simulink model "Wind_Turbine_Fixed_Speed_AC_to_DC_Output"  (R2019b)
settings: Solver=ode4  StartTime=0.0  StopTime=10  FixedStep=10e-6  RelTol=1e-3
libraries: powerlib x16, powerlib_meascontrol x5, re_lib x1, simulink x1
settings Model: Creator=KUNAL  LastModifiedBy=KUNAL

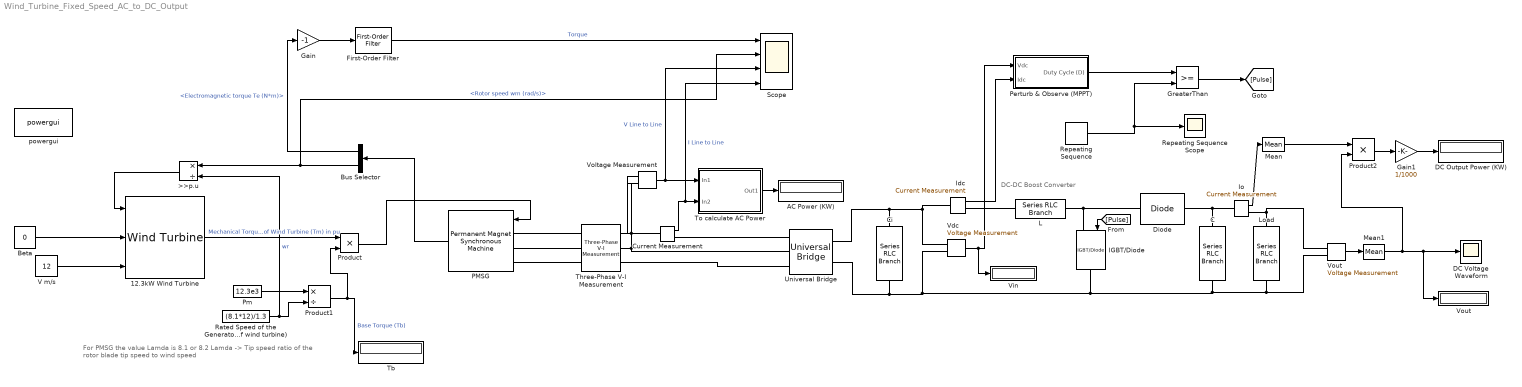
== system Wind_Turbine_Fixed_Speed_AC_to_DC_Output ==
  note: For PMSG the value Lamda is 8.1 or 8.2
      | Lamda -> Tip speed ratio of the rotor blade tip speed to wind speed
  note: DC-DC Boost Converter
  12.3kW Wind Turbine : re_lib/Wind Generation/Wind Turbine  Pnom=12.3e3  Pelec_base=12.3e3/0.9  wind_base=12  P_wind_base=0.85  speed_nom=1.2  pitch_angle=0  c1_c6="[0.51763          116          0.4            5           21     0.006795]"  cp_nom=0.48  lambda_nom=8.1
      settings: SourceProductName=Simscape Electrical  SourceProductBaseCode=PS
  ">>p.u " : Product  Inputs=*/
  "AC Power (KW) " : Display
  Beta : Constant  Value=0
  Bus Selector : BusSelector  OutputSignals=Electromagnetic torque Te (N*m),Rotor speed wm (rad/s)
  C : powerlib/Elements/Series RLC Branch  LConnTagsString=__new0  RConnTagsString=__new0  BranchType=C  Resistance=0.005  Inductance=1e-3  SetiL0=off  InitialCurrent=0  Capacitance=6.6094e-04  Setx0=off  InitialVoltage=0  Measurements=None
      settings: SourceProductName=Simscape Electrical
  "Ci " : powerlib/Elements/Series RLC Branch  LConnTagsString=__new0  RConnTagsString=__new0  BranchType=RC  Resistance=0.005  Inductance=1e-3  SetiL0=off  InitialCurrent=0  Capacitance=500e-6  Setx0=off  InitialVoltage=0  Measurements=None
      settings: SourceProductName=Simscape Electrical
  Current Measurement : powerlib/Measurements/Current Measurement  PhasorSimulation=off  OutputType=Complex  PSBequivalent=0
      settings: SourceProductName=Simscape Electrical
  "DC Output Power (KW) " : Display
  "DC Voltage Waveform " : Scope
  Diode : powerlib/Power Electronics/Diode  Ron=0.001  Lon=0  Vf=0.8  IC=0  UseSnubber=0  Rs=inf  Cs=inf  Measurements=off
      settings: SourceProductName=Simscape Electrical
  First-Order Filter : powerlib_meascontrol/Filters/First-Order Filter  FilterType=Lowpass  Tc=10e-3  Ts=50e-6  Initialize=on  Vac_Init=[0, 0, 50]  Vdc_Init=0  PlotResponse=off  FreqRange="[0,  200,  1]"
      settings: SourceProductName=Simscape Electrical
  Gain : Gain  Gain=-1
  Gain1 : Gain  Gain=1/1000
  GreaterThan : RelationalOperator  OutDataTypeStr=boolean  RndMeth=Simplest
  IGBT/Diode : powerlib/Power Electronics/IGBT//Diode  Ron=1e-3  Rs=1e5  Cs=inf  Measurements=off
      settings: SourceProductName=Simscape Electrical
  "Idc " : powerlib/Measurements/Current Measurement  PhasorSimulation=off  OutputType=Complex  PSBequivalent=0
      settings: SourceProductName=Simscape Electrical
  "Io " : powerlib/Measurements/Current Measurement  PhasorSimulation=off  OutputType=Complex  PSBequivalent=0
      settings: SourceProductName=Simscape Electrical
  "L " : powerlib/Elements/Series RLC Branch  LConnTagsString=__new0  RConnTagsString=__new0  BranchType=L  Resistance=0.005  Inductance=4.5573e-05  SetiL0=off  InitialCurrent=0  Capacitance=500e-6  Setx0=off  InitialVoltage=0  Measurements=None
      settings: SourceProductName=Simscape Electrical
  Load : powerlib/Elements/Series RLC Branch  LConnTagsString=__new0  RConnTagsString=__new0  BranchType=R  Resistance=13.5  Inductance=1e-3  SetiL0=off  InitialCurrent=0  Capacitance=500e-6  Setx0=off  InitialVoltage=0  Measurements=None
      settings: SourceProductName=Simscape Electrical
  Mean : powerlib_meascontrol/Measurements/Mean  Freq=60  Vinit=0  Ts=50e-6
      settings: SourceProductName=Simscape Electrical
  Mean1 : powerlib_meascontrol/Measurements/Mean  Freq=60  Vinit=0  Ts=50e-6
      settings: SourceProductName=Simscape Electrical
  "PMSG " : powerlib/Machines/Permanent Magnet Synchronous Machine  NbPhases=3  FluxDistribution=Sinusoidal  RotorType=Salient-pole  MechanicalLoad=Torque Tm  PresetModel=No  ShowDetailedParameters=on  MeasurementBus=off  Resistance=0.0485  Inductance=8.5e-3  dqInductances=[0.395e-3,0.395e-3]  La=0.000395  MachineConstant=Flux linkage established by magnets (V.s)  Flux=0.1194  VoltageCst=86.6271  TorqueCst=0.7164  Flat=120  Mechanical=[0.0027 0.0004924 4 0]  PolePairs=4  InitialConditions=[0,0, 0,0]  InitialConditions5ph=[0 0 0 0 0 0]  RefAngle=90 degrees behind phase A axis (modified Park)  IterativeDiscreteModel=Trapezoidal non iterative  TsBlock=-1  TsPowergui=0
  "Perturb & Observe (MPPT) " : Subsystem
  "Pm " : Constant  Value=12.3e3
  Product : Product  Inputs=**
  Product1 : Product  Inputs=*/
  Product2 : Product
  Rated Speed of the Generator (Wr) (Lamda * Wind Speed /Radius of wind turbine) : Constant  Value=(8.1*12)/1.3
  Repeating Sequence : simulink/Sources/Repeating Sequence  rep_seq_t=[0 1/20000]  rep_seq_y=[0 0.9]
  Repeating Sequence Scope : Scope
  Scope : Scope  NumInputPorts=4
  Tb : Display
  Three-Phase V-I Measurement : powerlib/Measurements/Three-Phase V-I Measurement  VoltageMeasurement=no  SetLabelV=off  LabelV=Vabc  Vpu=off  VpuLL=off  CurrentMeasurement=no  SetLabelI=off  LabelI=Iabc  Ipu=off  Pbase=100e6  Vbase=500e3  OutputType=Complex  PhasorSimulation=off  PSBequivalent=0
      settings: SourceProductName=Simscape Electrical
  To calculate AC Power : Subsystem
  "Universal Bridge " : powerlib/Power Electronics/Universal Bridge  Arms=3  SnubberResistance=1e5  SnubberCapacitance=inf  Device=Diodes  Ron=1e-3  Lon=0  ForwardVoltages="[  0  0  ]"  ForwardVoltage=0  GTOparameters=[ 10e-6 , 20e-6 ]  IGBTparameters=[ 1e-6 , 2e-6 ]  Measurements=None  Measurements_2=None  converterType=Rectifier
      settings: SourceProductName=Simscape Electrical
  V m/s : Constant  Value=12
  "Vdc " : powerlib/Measurements/Voltage Measurement  PhasorSimulation=off  OutputType=Complex  PSBequivalent=0
      settings: SourceProductName=Simscape Electrical
  "Vin " : Display
      settings: Format=bank
  Voltage Measurement : powerlib/Measurements/Voltage Measurement  PhasorSimulation=off  OutputType=Complex  PSBequivalent=0
      settings: SourceProductName=Simscape Electrical
  "Vout " : powerlib/Measurements/Voltage Measurement  PhasorSimulation=off  OutputType=Complex  PSBequivalent=0
      settings: SourceProductName=Simscape Electrical
  "Vout " : Display
      settings: Format=bank
  powergui : powerlib/powergui  Priority=1  SimulationMode=Discrete  SampleTime=20e-6  frequency=60  Iterations=50  frequencyindice=0  Pbase=100e6  ErrMax=1e-4  UnitsV=kV  UnitsW=MW  buscounter=0  FunctionMessages=off  echomessages=off  EnableUseOfTLC=off  CurrentSourceSwitches=off  DisableSnubberDevices=off  DisableRonSwitches=off  DisableVfSwitches=off  DisplayEquations=off  AutomaticDiscreteSolvers=off  SolverType=Tustin/Backward Euler (TBE)  Interpol=off  ExternalGateDelay=off  methode=off  Ts=100  x0status=blocks  SPID=on  SwTol=0  HookPort=off  NonlinearTolerance=1e-4  nMaxIteration=100  ContinueOnMaxIteration=off  RestoreLinks=warning  ResistiveCurrentMeasurement=off  Frange=[0:2:500]  Ylog=off  Xlog=on  ShowGrid=off  save=off  variable=ZData  structure=0  ZoomFFT=off  StartTime=0.0  cycles=1  DisplayStyle=1  fundamental=60  FreqAxis=off  MaxFrequency=1000  frequencyindicesteady=1  RmsSteady=1  display=off
      settings: SourceProductName=Simscape Electrical
  wires:
  Beta/1 -> 12.3kW Wind Turbine/2
  V m/s/1 -> 12.3kW Wind Turbine/3
  12.3kW Wind Turbine/1 -> Product/1  "Mechanical Torque of Wind Turbine (Tm) in pu"
  "Pm "/1 -> Product1/1
  Rated Speed of the Generator (Wr) (Lamda * Wind Speed /Radius of wind turbine)/1 -> ">>p.u "/2, Product1/2  "wr"
  Product1/1 -> Tb/1, Product/2  "Base Torque (Tb)"
  Product/1 -> "PMSG "/1
  "PMSG "/1 -> Bus Selector/1
  Bus Selector/2 -> Scope/2, ">>p.u "/1  "<Rotor speed wm (rad/s)>"
  ">>p.u "/1 -> 12.3kW Wind Turbine/1
  First-Order Filter/1 -> Scope/1  "Torque"
  Bus Selector/1 -> Gain/1  "<Electromagnetic torque Te (N*m)>"
  Gain/1 -> First-Order Filter/1
  Voltage Measurement/1 -> Scope/3, To calculate AC Power/1(In1)  "V Line to Line"
  Current Measurement/1 -> Scope/4, To calculate AC Power/2(In2)  "I Line to Line"
  To calculate AC Power/1(Out1) -> "AC Power (KW) "/1
  "Vdc "/1 -> "Vin "/1, "Perturb & Observe (MPPT) "/1("Vdc ")
  "Idc "/1 -> "Perturb & Observe (MPPT) "/2("Idc ")
  "Perturb & Observe (MPPT) "/1(Duty Cycle (D)) -> GreaterThan/1
  Repeating Sequence/1 -> GreaterThan/2, Repeating Sequence Scope/1
  [Pulse] -> IGBT/Diode/1
  GreaterThan/1 -> [Pulse]
  "Io "/1 -> Mean/1
  "Vout "/1 -> Mean1/1
  Mean/1 -> Product2/1
  Mean1/1 -> "Vout "/1, "DC Voltage Waveform "/1, Product2/2
  Product2/1 -> Gain1/1
  Gain1/1 -> "DC Output Power (KW) "/1
  connections:
  Three-Phase V-I Measurement/LConn2 -- "PMSG "/LConn2
  Three-Phase V-I Measurement/LConn1 -- "PMSG "/LConn1
  Three-Phase V-I Measurement/LConn3 -- "PMSG "/LConn3
  Voltage Measurement/LConn1 -- Current Measurement/LConn1 -- Three-Phase V-I Measurement/RConn1
  "Universal Bridge "/LConn2 -- Voltage Measurement/LConn2 -- Three-Phase V-I Measurement/RConn2
  Three-Phase V-I Measurement/RConn3 -- "Universal Bridge "/LConn3
  Current Measurement/RConn1 -- "Universal Bridge "/LConn1
  "Ci "/LConn1 -- "Vdc "/LConn1 -- "Idc "/LConn1 -- "Universal Bridge "/RConn1
  "Ci "/RConn1 -- Load/RConn1 -- "Vout "/LConn2 -- C/RConn1 -- IGBT/Diode/RConn1 -- "Vdc "/LConn2 -- "Universal Bridge "/RConn2
  "L "/LConn1 -- "Idc "/RConn1
  "L "/RConn1 -- IGBT/Diode/LConn1 -- Diode/LConn1
  C/LConn1 -- Diode/RConn1 -- "Io "/LConn1
  Load/LConn1 -- "Io "/RConn1 -- "Vout "/LConn1

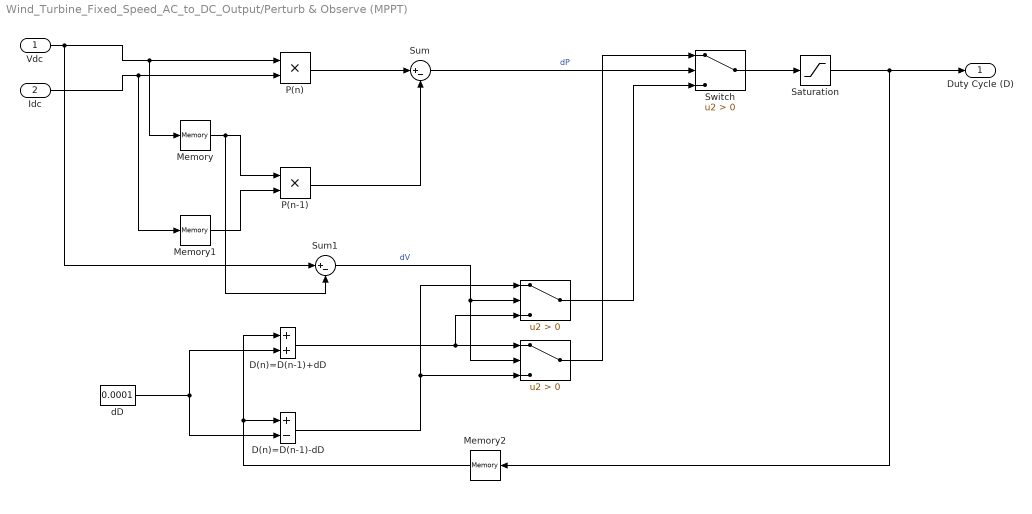
== system Wind_Turbine_Fixed_Speed_AC_to_DC_Output/Perturb & Observe (MPPT)  ==
  "Vdc " : Inport
  "Idc " : Inport  Port=2
  " " : Switch  Criteria=u2 > Threshold
  " " : Switch  Criteria=u2 > Threshold
  D(n)=D(n-1)+dD : Sum
  D(n)=D(n-1)-dD : Sum  Inputs=+-
  Memory : Memory
  Memory1 : Memory
  Memory2 : Memory
  "P(n) " : Product
  P(n-1) : Product
  Saturation : Saturate  UpperLimit=inf
  Sum : Sum  Inputs=|+-
  Sum1 : Sum  Inputs=|+-
  Switch : Switch  Criteria=u2 > Threshold
  dD : Constant  Value=0.0001
  Duty Cycle (D) : Outport
  wires:
  "Vdc "/1 -> Sum1/1, Memory/1, "P(n) "/1
  "Idc "/1 -> Memory1/1, "P(n) "/2
  Memory/1 -> Sum1/2, P(n-1)/1
  Memory1/1 -> P(n-1)/2
  "P(n) "/1 -> Sum/1
  P(n-1)/1 -> Sum/2
  Sum/1 -> Switch/2  "dP"
  Switch/1 -> Saturation/1
  Memory2/1 -> D(n)=D(n-1)-dD/1, D(n)=D(n-1)+dD/1
  dD/1 -> D(n)=D(n-1)-dD/2, D(n)=D(n-1)+dD/2
  D(n)=D(n-1)-dD/1 -> " "/1, " "/3
  D(n)=D(n-1)+dD/1 -> " "/3, " "/1
  Sum1/1 -> " "/2, " "/2  "dV"
  " "/1 -> Switch/3
  " "/1 -> Switch/1
  Saturation/1 -> Memory2/1, Duty Cycle (D)/1

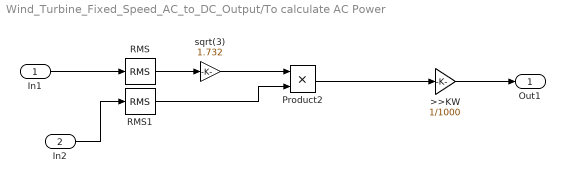
== system Wind_Turbine_Fixed_Speed_AC_to_DC_Output/To calculate AC Power ==
  In1 : Inport
  In2 : Inport  Port=2
  ">>KW " : Gain  Gain=1/1000
  Product2 : Product  Inputs=**
  RMS : powerlib_meascontrol/Measurements/RMS  TrueRMS=on  Freq=50  RMSInit=120  Ts=50e-6
      settings: SourceProductName=Simscape Electrical
  RMS1 : powerlib_meascontrol/Measurements/RMS  TrueRMS=on  Freq=50  RMSInit=120  Ts=50e-6
      settings: SourceProductName=Simscape Electrical
  "sqrt(3) " : Gain  Gain=1.732
  Out1 : Outport
  wires:
  "sqrt(3) "/1 -> Product2/1
  RMS/1 -> "sqrt(3) "/1
  RMS1/1 -> Product2/2
  In1/1 -> RMS/1
  In2/1 -> RMS1/1
  ">>KW "/1 -> Out1/1
  Product2/1 -> ">>KW "/1
